simulink model "hinf_control_with_integrator_multimodel_open_loop_system"  (R2020b)
settings: Solver=VariableStepAuto  StartTime=0.0  StopTime=200  RelTol=1e-3
values from neighbouring files (symbols this model uses):
  COUPLING_COEFFICIENT = 0.5736    [Workshop_MATLAB.m]
  ESTIMATOR_TRANSFER_FUNCTION_DENOMINATOR = [ESTIMATOR_TIME_CONSTANT 1]    [Workshop_MATLAB.m]
  ESTIMATOR_TRANSFER_FUNCTION_NUMERATOR = [1 0]    [Workshop_MATLAB.m]
  FLEXIBLE_MODE_DAMPING_RATIO = 0.00495    [Workshop_MATLAB.m]
  FLEXIBLE_MODE_FREQUENCY = 2.6268    [Workshop_MATLAB.m]
  INITIAL_CONDITION_ON_STATE = 0.0001    [Workshop_MATLAB.m]
  REACTION_WHEEL_DYNAMICS_DENOMINATOR = [1 2.400 0.763]    [Workshop_MATLAB.m]
  REACTION_WHEEL_DYNAMICS_NUMERATOR = REACTION_WHEEL_INERTIA*[1.214 0.763 0]    [Workshop_MATLAB.m]
  REACTION_WHEEL_INERTIA = 0.0004    [Workshop_MATLAB.m]
undefined symbols (not defined in the file or in its folder): differenceToSecondOrderWithIntegratorMultimodalWeightStateSpace, positionWithIntegratorMultimodalWeightStateSpace, satelliteInertia, TARGET_SECOND_ORDER, torqueWithIntegratorMultimodalWeightStateSpace
settings Model: Creator=WLCG  LastModifiedBy=WLCG

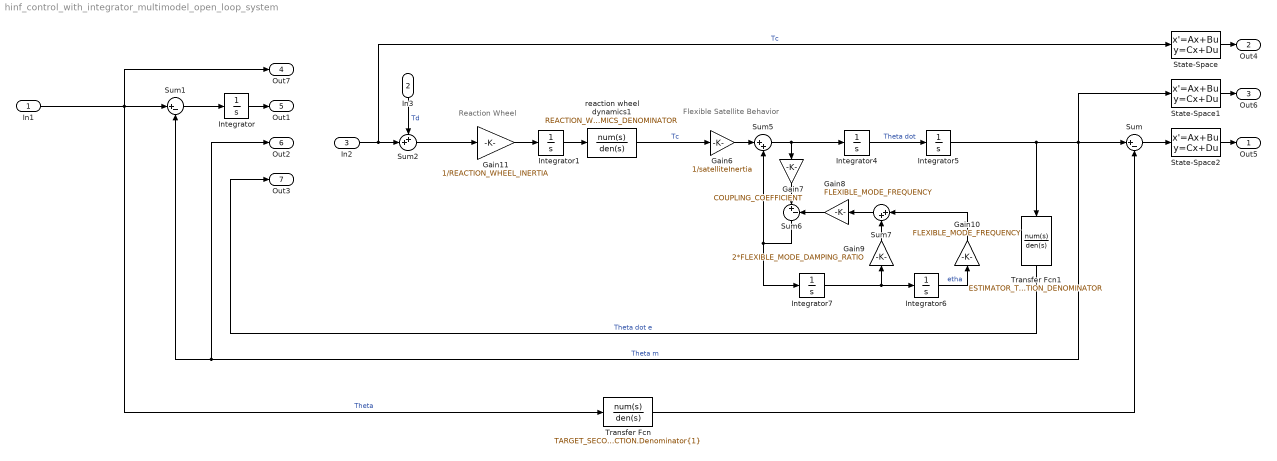
== system hinf_control_with_integrator_multimodel_open_loop_system ==
  note: Flexible Satellite Behavior
  note: Reaction Wheel
  In1 : Inport
  In3 : Inport  Port=2
  In2 : Inport  Port=3
  Gain10 : Gain  Gain=FLEXIBLE_MODE_FREQUENCY
  Gain11 : Gain  Gain=1/REACTION_WHEEL_INERTIA
  Gain6 : Gain  Gain=1/satelliteInertia
  Gain7 : Gain  Gain=COUPLING_COEFFICIENT
  Gain8 : Gain  Gain=FLEXIBLE_MODE_FREQUENCY
  Gain9 : Gain  Gain=2*FLEXIBLE_MODE_DAMPING_RATIO
  Integrator{,1,4..5,7} (5 alike) : Integrator
  Integrator6 : Integrator  InitialCondition=INITIAL_CONDITION_ON_STATE
  State-Space : StateSpace  A=torqueWithIntegratorMultimodalWeightStateSpace.A  B=torqueWithIntegratorMultimodalWeightStateSpace.B  C=torqueWithIntegratorMultimodalWeightStateSpace.C  D=torqueWithIntegratorMultimodalWeightStateSpace.D  InitialCondition=0
  State-Space1 : StateSpace  A=positionWithIntegratorMultimodalWeightStateSpace.A  B=positionWithIntegratorMultimodalWeightStateSpace.B  C=positionWithIntegratorMultimodalWeightStateSpace.C  D=positionWithIntegratorMultimodalWeightStateSpace.D  InitialCondition=0
  State-Space2 : StateSpace  A=differenceToSecondOrderWithIntegratorMultimodalWeightStateSpace.A  B=differenceToSecondOrderWithIntegratorMultimodalWeightStateSpace.B  C=differenceToSecondOrderWithIntegratorMultimodalWeightStateSpace.C  D=differenceToSecondOrderWithIntegratorMultimodalWeightStateSpace.D  InitialCondition=0
  Sum : Sum  Inputs=|+-
  Sum1 : Sum  Inputs=|+-
  Sum2 : Sum  Inputs=++|
  Sum5 : Sum  Inputs=|++
  Sum6 : Sum  Inputs=|+-
  Sum7 : Sum  Inputs=|++
  Transfer Fcn : TransferFcn  Numerator=TARGET_SECOND_ORDER.TRANSFER_FUNCTION.Numerator{1}  Denominator=TARGET_SECOND_ORDER.TRANSFER_FUNCTION.Denominator{1}
  Transfer Fcn1 : TransferFcn  Numerator=ESTIMATOR_TRANSFER_FUNCTION_NUMERATOR  Denominator=ESTIMATOR_TRANSFER_FUNCTION_DENOMINATOR
  reaction wheel dynamics1 : TransferFcn  Numerator=REACTION_WHEEL_DYNAMICS_NUMERATOR  Denominator=REACTION_WHEEL_DYNAMICS_DENOMINATOR
  Out5 : Outport
  Out4 : Outport  Port=2
  Out6 : Outport  Port=3
  Out7 : Outport  Port=4
  Out1 : Outport  Port=5
  Out2 : Outport  Port=6
  Out3 : Outport  Port=7
  wires:
  Gain7/1 -> Sum6/1
  Gain9/1 -> Sum7/2
  Sum7/1 -> Gain8/1
  Integrator5/1 -> State-Space1/1, Sum1/2, Out2/1, Sum/1, Transfer Fcn1/1  "Theta m"
  Gain10/1 -> Sum7/1
  reaction wheel dynamics1/1 -> Gain6/1  "Tc"
  Gain8/1 -> Sum6/2
  Integrator4/1 -> Integrator5/1  "Theta dot"
  Gain6/1 -> Sum5/1
  Gain11/1 -> Integrator1/1
  Sum5/1 -> Integrator4/1, Gain7/1
  Integrator6/1 -> Gain10/1  "etha"
  Integrator7/1 -> Integrator6/1, Gain9/1
  Integrator1/1 -> reaction wheel dynamics1/1
  Sum6/1 -> Integrator7/1, Sum5/2
  Transfer Fcn1/1 -> Out3/1  "Theta dot e"
  In1/1 -> Sum1/1, Out7/1, Transfer Fcn/1  "Theta"
  Transfer Fcn/1 -> Sum/2
  Sum/1 -> State-Space2/1
  State-Space2/1 -> Out5/1
  Integrator/1 -> Out1/1
  Sum1/1 -> Integrator/1
  Sum2/1 -> Gain11/1
  In2/1 -> Sum2/2, State-Space/1  "Tc"
  In3/1 -> Sum2/1  "Td"
  State-Space1/1 -> Out6/1
  State-Space/1 -> Out4/1
